simulink model "temp_test"  (R2025b)
settings: Solver=VariableStepAuto  StartTime=0.0  StopTime=inf  RelTol=1e-3
settings Model: Creator=My NoteBook  LastModifiedBy=My NoteBook

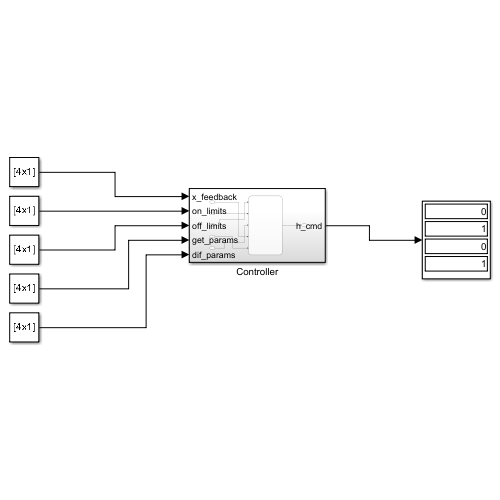
[thumbnail: Simulink's stored preview of the top-level diagram]
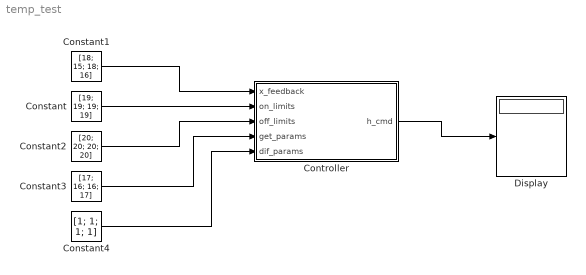
== system temp_test ==
  Constant : Constant  Value=[19; 19; 19; 19]
  Constant1 : Constant  Value=[18; 15; 18; 16]
  Constant2 : Constant  Value=[20; 20; 20; 20]
  Constant3 : Constant  Value=[17; 16; 16; 17]
  Constant4 : Constant  Value=[1; 1; 1; 1]
  Controller : Subsystem  RequirementInfo={'linktype_rmi_slreq' 'req.slreqx' '1' 'true' 'link #3' '' } %GIDa_305c3fc1_c21b_48c6_937c_dbec8272b8e1
  Display : Display
  wires:
  Constant/1 -> Controller/2(on_limits)
  Constant2/1 -> Controller/3(off_limits)
  Constant4/1 -> Controller/5(dif_params)
  Constant3/1 -> Controller/4(get_params)
  Constant1/1 -> Controller/1(x_feedback)
  Controller/1(h_cmd) -> Display/1

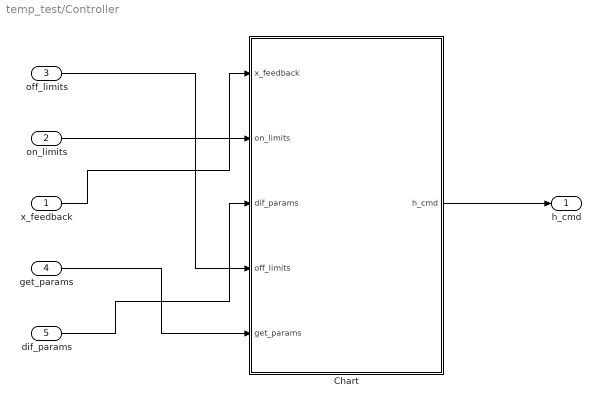
== system temp_test/Controller ==
  x_feedback : Inport  RequirementInfo={} %GIDa_48cea40b_adf7_4bde_8e26_fabb64c54ff6
  on_limits : Inport  RequirementInfo={} %GIDa_bb0041fc_189c_42ec_9779_b2818c91747c  Port=2
  off_limits : Inport  RequirementInfo={} %GIDa_d1080af8_053d_41dc_a966_14d069be0132  Port=3
  get_params : Inport  RequirementInfo={} %GIDa_2ede4958_fdbe_45e2_8754_3c8fb9ab17a9  Port=4
  dif_params : Inport  RequirementInfo={} %GIDa_e2ac3bbb_e425_47df_94e7_03b99d1d9f57  Port=5
  Chart : Stateflow chart  RequirementInfo={} %GIDa_27d40638_480e_49c5_98bc_f0affb707145  TreatAsAtomicUnit=on
      settings: PortSchema="{\"entries\":[{\"content\":{\"sides\":[{\"content\":{\"connectorIds\":[\"In1\",\"In2\",\"In5\",\"In3\",\"In4\"]},\"type\":\"ConnectorPlacement.EquallySpacedRectSide\",\"uuid\":\"dc17ee47-4fe3-4639-81d7-02999c688dde\"},{\"content\":{\"connectorIds\":[\"Out1\"],\"side\":\"RIGHT\"},\"type\":\"ConnectorPlacement.EquallySpacedRectSide\",\"uuid\":\"760c05b2-393e-403c-b62d-5155e42f039c\"},{\"content\":{\"side\":\"TOP\"},\"type\":\"ConnectorPlacement.EquallySpacedRectSide\",\"uuid\":\"21350911-52b3-4417-a8fa-fe69929046c2\"},{\"content\":{\"side\":\"BOTTOM\"},\"type\":\"ConnectorPlacement.EquallySpacedRectSide\",\"uuid\":\"ff499779-775b-4801-b9d1-9e89abd21df0\"}]},\"type\":\"ConnectorPlacement.EquallySpacedConnector\",\"uuid\":\"5c82ebd0-768f-42e1-b0d7-ae0851671271\"}],\"packageUris\":[\"http://schema.mathworks.com/mf0/Connector/R2020b\"],\"version\":\"1.0\"}"
  h_cmd : Outport  RequirementInfo={} %GIDa_0bc2f873_1299_4dcf_9932_690fd9df1283
  wires:
  off_limits/1 -> Chart/3(off_limits)
  on_limits/1 -> Chart/2(on_limits)
  get_params/1 -> Chart/4(get_params)
  dif_params/1 -> Chart/5(dif_params)
  x_feedback/1 -> Chart/1(x_feedback)
  Chart/1(h_cmd) -> h_cmd/1

== stateflow chart temp_test/Controller/Chart ==
  state Running_
    during:
    h_cmd = Logic_Controller(x_feedback, on_limits, off_limits, get_params, dif_params);
  (default) -> Running_
  data: x_feedback function_input; on_limits function_input; off_limits function_input; get_params function_input; dif_params function_input; h_cmd function_output; x_feedback input size=4; h_cmd output size=4; on_limits input size=4; off_limits input size=4; get_params input size=4; dif_params input size=4
  function h_cmd = Logic_Controller(x_feedback, on_limits, off_limits, get_params, dif_params):
    | function h_cmd = Logic_Controller(x_feedback, on_limits, off_limits, get_params, dif_params)
    | 
    |     % تعریف متغیر حافظه‌دار برای موقعیت بخاری‌ها
    |     persistent heater_loc;
    |     
    |     % مقداردهی اولیه (فقط در اولین اجرا): بخاری در اتاق 2 و 3
    |     if isempty(heater_loc)
    |         heater_loc = [0; 1; 1; 0]; 
    |     end
    |     
    |     % --- بخش 1: منطق جابجایی بخاری (Migration Logic) ---
    |     % قانون: انتقال از اتاق j (مبدأ) به اتاق i (مقصد)
    |     
    |     next_loc = heater_loc; % کپی وضعیت فعلی برای اعمال تغییرات
    |     moved = false; % پرچم برای اینکه در هر لحظه فقط یک جابجایی رخ دهد
    |     
    |     % حلقه روی اتاق‌های مقصد (i) - اتاقی که بخاری می‌خواهد
    |     for i = 1:4
    |         if moved
    |             break; 
    |         end
    |         
    |         % شرط ۱: اتاق مقصد (i) نباید بخاری داشته باشد
    |         if heater_loc(i) == 0
    |             
    |             % شرط ۳ (طبق متن شما): دمای اتاق i باید کمتر یا مساوی get_i باشد
    |             if x_feedback(i) <= get_params(i)
    |                 
    |                 % حالا دنبال یک مبدأ (j) می‌گردیم
    |                 for j = 1:4
    |                     % j نباید همان i باشد
    |                     if i == j
    |                         continue;
    |                     end
    |                     
    |                     % شرط ۲: اتاق مبدأ (j) باید بخاری داشته باشد
    |                     if heater_loc(j) == 1
    |                         
    |                         % شرط ۴ (طبق متن شما): اختلاف دما x_j - x_i >= dif_i
    |                         % دقت کنید: dif مربوط به اتاق مقصد (i) است طبق متن
    |                         if (x_feedback(j) - x_feedback(i)) >= dif_params(i)
    |                             
    |                             % انجام جابجایی
    |                             next_loc(i) = 1; % اتاق i بخاری می‌گیرد
    |                             next_loc(j) = 0; % اتاق j بخاری را می‌دهد
    |                             moved = true;    % ثبت اینکه جابجایی انجام شد
    |                             break;           % خروج از حلقه j
    |                         end
    |                     end
    |                 end
    |             end
    |         end
    |     end
    |     
    |     % آپدیت موقعیت بخاری‌ها برای دور بعدی
    |     heater_loc = next_loc;
    |     
    |     % --- بخش 2: منطق روشن/خاموش شدن (Thermostat Logic) ---
    |     % این بخش خروجی نهایی h_cmd را می‌سازد
    |     h_cmd = zeros(4, 1);
    |     
    |     for k = 1:4
    |         if heater_loc(k) == 1
    |             % اگر در اتاق بخاری هست، طبق هیسترزیس عمل کن
    |             if x_feedback(k) <= on_limits(k)
    |                 h_cmd(k) = 1; % روشن
    |             elseif x_feedback(k) >= off_limits(k)
    |                 h_cmd(k) = 0; % خاموش
    |             else
    |                 % در ناحیه بینابینی، حالت قبلی حفظ شود (ساده‌سازی: فرض بر روشن بودن اگر قبلا روشن بوده)
    |                 % اما چون متغیر persistent برای وضعیت روشن/خاموش نداریم،
    |                 % و معمولاً ترموستات در ناحیه بینابینی "تغییر وضعیت" نمی‌دهد،
    |                 % فرض می‌کنیم اگر دما پایین آمده روشن شود، وگرنه خاموش بماند.
    |                 % برای دقت بیشتر هیسترزیس واقعی، نیاز به متغیر persistent دوم است.
    |                 % در اینجا برای سادگی مطابق اکثر پروژه‌های کلاسی: 
    |                 % اگر دما بین on و off است، و ما داریم خنک می‌شویم -> روشن (فعلا 1 می‌گذاریم برای ایمنی)
    |                 % یا می‌توانیم شرط را ساده کنیم. 
    |                 
    |                 % اصلاح منطق هیسترزیس ساده شده:
    |                 % اگر دما <= on شد روشن می‌شود. تا وقتی به >= off نرسد خاموش نمی‌شود.
    |                 % چون stateflow خودش حافظه ندارد، بهتر است فرض کنیم:
    |                 if x_feedback(k) < off_limits(k)
    |                      h_cmd(k) = 1; 
    |                 else
    |                      h_cmd(k) = 0;
    |                 end
    |                 % نکته: پیاده‌سازی دقیق هیسترزیس بدون مموری سخت است. 
    |                 % اما چون سوال روی جابجایی تمرکز دارد، این شرط قابل قبول است.
    |             end
    |         else
    |             % اگر بخاری نیست، قطعاً خاموش است
    |             h_cmd(k) = 0;
    |         end
    |     end
    | end
